simulink model "MCS"  (R2022b)
settings: Solver=FixedStepAuto  StartTime=0.0  StopTime=inf  RelTol=1e-3  EnableMultiTasking=on
undefined symbols (not defined in the file or in its folder): CR, INPUT, LF, MCS_SAMPLING_TIME, SAMPLING_TIME
libraries: instrumentseriallib x2, sharedtransform x2, aerolibanimutils x1, instrumentlib x1
Description:
  | Packet Input/Output
  | 
  | The example model "sldrtex_packetio" shows how to transfer data through
  | UDP communication protocol using binary encoding. The model sends data
  | within one computer, from one UDP port to another. You can modify the
  | model to communicate between two computers by splitting this model
  | into its send and receive parts and running the models on two computers.
  | The yellow blocks are used to send the data, the blue blocks
  | are used to receive the data. Then, please enter the host names or
  | IP addresses of the two computers into the appropriate fields
  | in the Board Setup dialog.
  | 
  | How to run this model in Normal Mode:
  | 
  | 1) Double-click the orange button to switch to Normal Mode if needed.
  | 2) Start the real-time execution using Simulation->Run.
  | 
  | How to run this model in External Mode:
  | 
  | 1) Double-click the orange button to switch to External Mode if needed.
  | 2) Start the real-time execution using Simulation->Run. The model will automatically
  |    build, connect to Simulink in External Mode and start.
settings Model: ExtModeTrigDuration=12000  Creator=The MathWorks, Inc.  LastModifiedBy=drones
settings SolverCC: AlgebraicLoopSolver=TrustRegion
settings DataIOCC: LimitDataPoints=on  SaveFormat=Array  SignalLoggingSaveFormat=ModelDataLogs  ReturnWorkspaceOutputs=off
settings OptimizationCC: ExpressionDepthLimit=2147483647  InitFltsAndDblsToZero=on  EfficientMapNaN2IntZero=off
settings DebuggingCC: MergeDetectMultiDrivingBlocksExec=none  SolverPrmCheckMsg=warning  MultiTaskDSMMsg=none  FcnCallInpInsideContextMsg=warning  UnconnectedInputMsg=warning  UnconnectedOutputMsg=warning  UnconnectedLineMsg=warning  AllowSymbolicDim=off  StateNameClashWarn=warning  SFUnexpectedBacktrackingDiag=warning  SFNoUnconditionalDefaultTransitionDiag=warning  SFExecutionAtInitializationDiag=none  SFMachineParentedDataDiag=warning  ArithmeticOperatorsInVariantConditions=warning
settings HardwareCC: ProdBitPerLong=64  ProdHWDeviceType=Intel->x86-64 (Linux 64)
settings ModelReferenceCC: EnableRefExpFcnMdlSchedulingChecks=on  PropagateSignalLabelsOutOfModel=off
settings SFSimCC: SimUseLocalCustomCode=off  CustomCodeUndefinedFunction=UseInterfaceOnly
settings RTWCC: Description=Simulink Desktop Real-Time  SystemTargetFile=sldrt.tlc  TemplateMakefile=sldrt.tmf  RTWUseLocalCustomCode=off  RTWCompilerOptimization=on  DLArmComputeVersion=19.05
settings CodeAppCC: MaxIdLength=95  StateflowObjectComments=on
settings SimulinkDesktopRealTimeCC: TargetLibSuffix=_sldrt.a  TargetPreCompLibLocation=C:\Program Files\MATLAB\R2022b\toolbox\sldrt\lib\win64  TargetLangStandard=C89/C90 (ANSI)
settings ConfigComp: CovMetricSettings=dsw  CovSaveCumulativeToWorkspaceVar=on  CovSaveSingleToWorkspaceVar=on  CovExternalEMLEnable=off

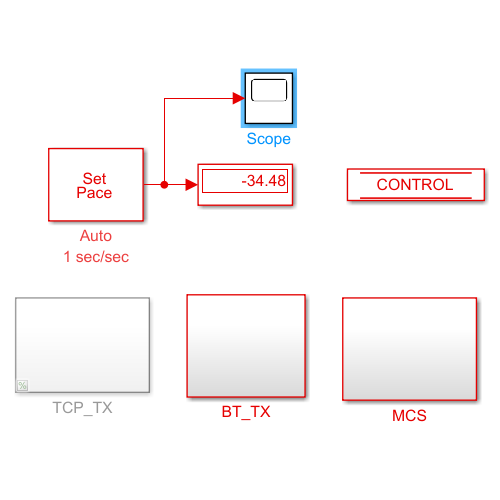
[thumbnail: Simulink's stored preview of the top-level diagram]
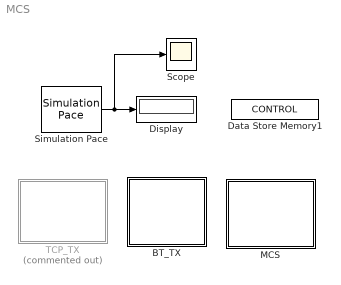
== system MCS ==
  BT_TX : Subsystem
  Data Store Memory1 : DataStoreMemory  Priority=2  DataStoreName=CONTROL  ReadBeforeWriteMsg=warning  WriteAfterWriteMsg=warning  WriteAfterReadMsg=warning  InitialValue=CONTROL_INI  ShowAdditionalParam=off  OutDataTypeStr=Bus: CONTROL_Bus
  Display : Display
  MCS : Subsystem
  Scope : Scope
  Simulation Pace : aerolibanimutils/Simulation Pace  SimulationPace=1  SleepMode=Auto  OutputPaceError=on  SampleTime=MCS_SAMPLING_TIME
  TCP_TX : Subsystem  Commented=on
  wires:
  Simulation Pace/1 -> Scope/1, Display/1

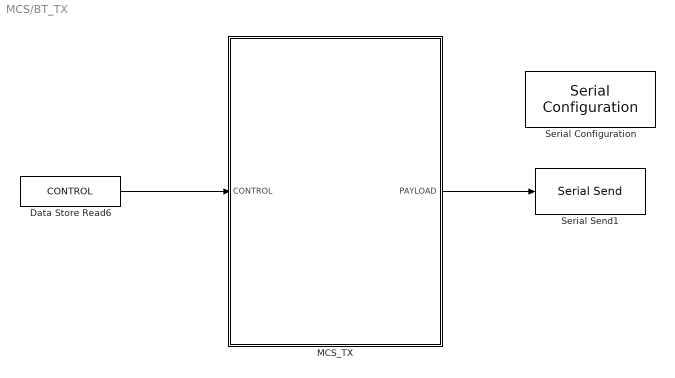
== system MCS/BT_TX ==
  Data Store Read6 : DataStoreRead  DataStoreName=CONTROL  SampleTime=SAMPLING_TIME  IndexOptions=Index vector (dialog)  Indices=1  OutputSizes=1
  MCS_TX : MATLAB Function  Priority=20  TreatAsAtomicUnit=on
  Serial Configuration : instrumentseriallib/Serial Configuration  Priority=-200000  PortSel=COM3  Port=COM3  ComPort=COM3  BaudRate=115200  DataBits=8  Parity=none  StopBits=1  ByteOrder=little-endian  FlowControl=none  Timeout=10e-3  SimulateUsing=Interpreted execution  BlockInModel=on  aMode=1
  Serial Send1 : instrumentseriallib/Serial Send  PortSel=COM3  Port=COM3  ComPort=COM3  Header=[254 ]  Terminator=CR/LF ('\r\n')  CustomTerminator=[]  EnableBlockingMode=off  SimulateUsing=Interpreted execution  BlockInModel=on  aMode=1
  wires:
  Data Store Read6/1 -> MCS_TX/1(CONTROL)
  MCS_TX/1(PAYLOAD) -> Serial Send1/1

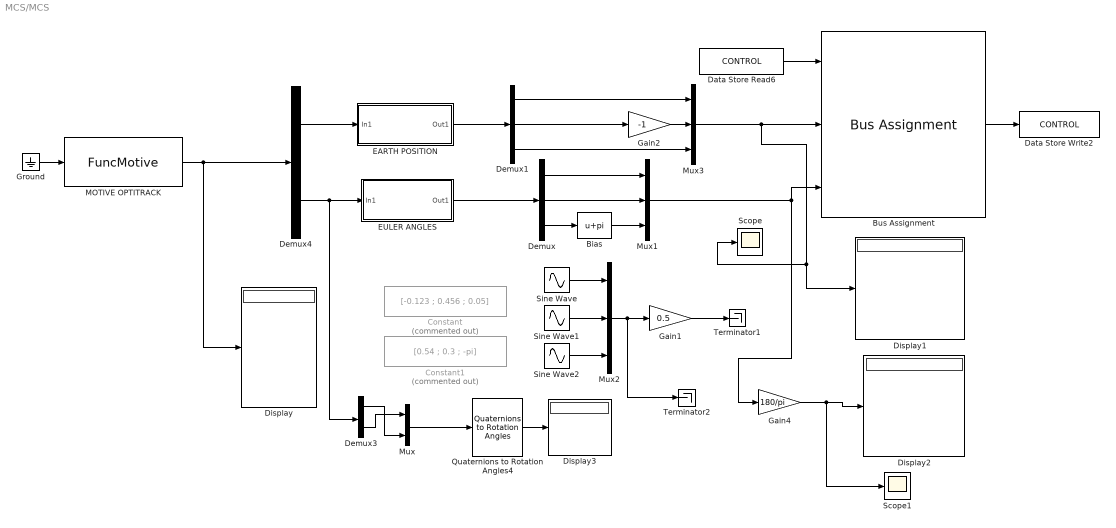
== system MCS/MCS ==
  Bias : Bias  Bias=pi  SaturateOnIntegerOverflow=off
  Bus Assignment : BusAssignment  AssignedSignals=INPUT.MCS_EARTH_POS,INPUT.MCS_EULER_ANG
  Constant : Constant  Commented=on  Value=[-0.123 ; 0.456 ; 0.05]  SampleTime=SAMPLING_TIME
  Constant1 : Constant  Commented=on  Value=[0.54 ; 0.3 ; -pi]  SampleTime=SAMPLING_TIME
  Data Store Read6 : DataStoreRead  DataStoreName=CONTROL  SampleTime=MCS_SAMPLING_TIME  IndexOptions=Index vector (dialog)  Indices=1  OutputSizes=1
  Data Store Write2 : DataStoreWrite  DataStoreName=CONTROL  IndexOptions=Index vector (dialog)  Indices=1  OutputSizes=1
  Demux : Demux  Outputs=3
  Demux1 : Demux  Outputs=3
  Demux3 : Demux  Outputs=[1 -1]
  Demux4 : Demux  Outputs=[3 4]
  Display{,1..3} (4 alike) : Display
  EARTH POSITION : Subsystem
  EULER ANGLES : Subsystem
  Gain1 : Gain  Gain=0.5
  Gain2 : Gain  Gain=-1
  Gain4 : Gain  Gain=180/pi
  Ground : Ground
  MOTIVE OPTITRACK : M-S-Function  FunctionName=FuncMotive  Parameters=1
  Mux : Mux  Inputs=2
  Mux1 : Mux  Inputs=3
  Mux2 : Mux  Inputs=3
  Mux3 : Mux  Inputs=3
  Quaternions to Rotation Angles4 : sharedtransform/Quaternions to Rotation Angles  rotationOrder=YZX  aMode=aMode
  Scope : Scope
  Scope1 : Scope
  Sine Wave : Sin  SineType=Sample based  Amplitude=2  Bias=0.5  Samples=360  SampleTime=MCS_SAMPLING_TIME
  Sine Wave1 : Sin  SineType=Sample based  Amplitude=2  Bias=0.5  Samples=360  SampleTime=MCS_SAMPLING_TIME  Offset=60
  Sine Wave2 : Sin  SineType=Sample based  Amplitude=2  Bias=0.5  Samples=360  SampleTime=MCS_SAMPLING_TIME  Offset=120
  Terminator1 : Terminator
  Terminator2 : Terminator
  wires:
  Ground/1 -> MOTIVE OPTITRACK/1
  Demux4/2 -> Demux3/1, EULER ANGLES/1(In1)
  Demux4/1 -> EARTH POSITION/1(In1)
  Data Store Read6/1 -> Bus Assignment/1
  Bus Assignment/1 -> Data Store Write2/1
  MOTIVE OPTITRACK/1 -> Display/1, Demux4/1
  Demux3/2 -> Mux/1
  Mux/1 -> Quaternions to Rotation Angles4/1
  Quaternions to Rotation Angles4/1 -> Display3/1
  Demux3/1 -> Mux/2
  Demux/3 -> Bias/1
  Bias/1 -> Mux1/3
  Demux/2 -> Mux1/2
  Demux/1 -> Mux1/1
  EULER ANGLES/1(Out1) -> Demux/1
  Sine Wave/1 -> Mux2/1
  Sine Wave1/1 -> Mux2/2
  Sine Wave2/1 -> Mux2/3
  Mux2/1 -> Terminator2/1, Gain1/1
  Gain4/1 -> Scope1/1, Display2/1
  EARTH POSITION/1(Out1) -> Demux1/1
  Gain1/1 -> Terminator1/1
  Mux1/1 -> Gain4/1, Bus Assignment/3
  Mux3/1 -> Scope/1, Display1/1, Bus Assignment/2
  Demux1/1 -> Mux3/1
  Demux1/2 -> Gain2/1
  Gain2/1 -> Mux3/2
  Demux1/3 -> Mux3/3

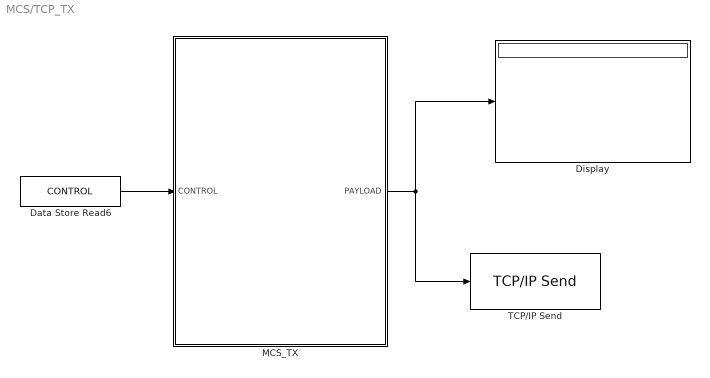
== system MCS/TCP_TX ==
  Data Store Read6 : DataStoreRead  DataStoreName=CONTROL  SampleTime=MCS_SAMPLING_TIME  IndexOptions=Index vector (dialog)  Indices=1  OutputSizes=1
  Display : Display
  MCS_TX : MATLAB Function  Priority=20  TreatAsAtomicUnit=on
  TCP/IP Send : instrumentlib/TCP//IP Send  Host=192.168.0.107  Port=15000  ByteOrder=big-endian  EnableBlockingMode=off  Timeout=SAMPLING_TIME  TransferDelay=off  SimulateUsing=Interpreted execution
  wires:
  MCS_TX/1(PAYLOAD) -> TCP/IP Send/1, Display/1
  Data Store Read6/1 -> MCS_TX/1(CONTROL)

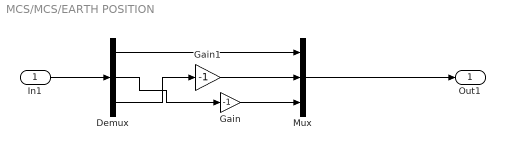
== system MCS/MCS/EARTH POSITION ==
  In1 : Inport
  Demux : Demux  Outputs=3
  Gain : Gain  Gain=-1
  Gain1 : Gain  Gain=-1
  Mux : Mux  Inputs=3
  Out1 : Outport  VectorParamsAs1DForOutWhenUnconnected=off
  wires:
  In1/1 -> Demux/1
  Demux/1 -> Mux/1
  Demux/2 -> Gain/1
  Demux/3 -> Gain1/1
  Mux/1 -> Out1/1
  Gain/1 -> Mux/3
  Gain1/1 -> Mux/2

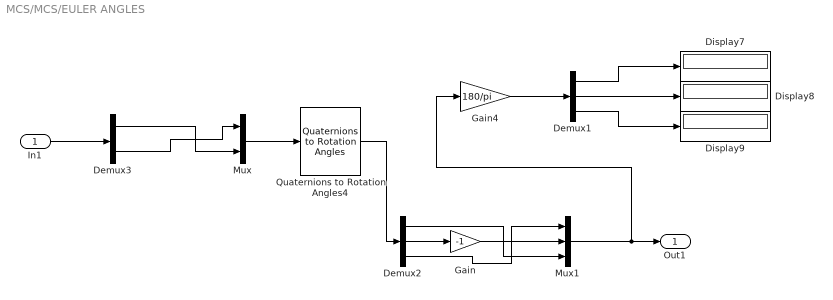
== system MCS/MCS/EULER ANGLES ==
  In1 : Inport
  Demux1 : Demux  Outputs=3
  Demux2 : Demux  Outputs=3
  Demux3 : Demux  Outputs=[1 -1]
  Display7 : Display
  Display8 : Display
  Display9 : Display
  Gain : Gain  Gain=-1
  Gain4 : Gain  Gain=180/pi
  Mux : Mux  Inputs=2
  Mux1 : Mux  Inputs=3
  Quaternions to Rotation Angles4 : sharedtransform/Quaternions to Rotation Angles  rotationOrder=YZX  aMode=aMode
  Out1 : Outport  VectorParamsAs1DForOutWhenUnconnected=off
  wires:
  Mux/1 -> Quaternions to Rotation Angles4/1
  Demux1/1 -> Display7/1
  Quaternions to Rotation Angles4/1 -> Demux2/1
  Demux1/3 -> Display9/1
  Demux1/2 -> Display8/1
  In1/1 -> Demux3/1
  Demux3/1 -> Mux/2
  Demux3/2 -> Mux/1
  Demux2/1 -> Mux1/3
  Mux1/1 -> Gain4/1, Out1/1
  Gain4/1 -> Demux1/1
  Demux2/3 -> Mux1/1
  Demux2/2 -> Gain/1
  Gain/1 -> Mux1/2

== matlab function MCS/TCP_TX/MCS_TX ==
  data: CONTROL input; PAYLOAD output uint8 size=26
function PAYLOAD = MCS_TX(CONTROL)

% Payload definition
PAYLOAD = [typecast(single(CONTROL.INPUT.MCS_EARTH_POS(1)),'uint8')'
    typecast(single(CONTROL.INPUT.MCS_EARTH_POS(2)),'uint8')'
    typecast(single(CONTROL.INPUT.MCS_EARTH_POS(3)),'uint8')'
    typecast(single(CONTROL.INPUT.MCS_EULER_ANG(1)),'uint8')'
    typecast(single(CONTROL.INPUT.MCS_EULER_ANG(2)),'uint8')'
    typecast(single(CONTROL.INPUT.MCS_EULER_ANG(3)),'uint8')'
    uint8(0) ; uint8(0)];
% CRC computation
CRC_VALUE = uint16(65535);
for nn=1:length(PAYLOAD)-2
    TMP = bitxor(uint16(PAYLOAD(nn)),bitand(CRC_VALUE,uint16(255)));
    TMP4 = bitand(bitshift(TMP,4),uint16(255));
    TMP = bitxor(TMP,TMP4);
    TMP8 = bitshift(TMP,8);
    TMP3 = bitshift(TMP,3);
    TMP_4 = bitshift(TMP,-4); 
    CRC_VALUE = bitxor(bitshift(CRC_VALUE,-8),bitxor(TMP8,bitxor(TMP3,TMP_4)));
    CRC_VALUE = bitand(CRC_VALUE,uint16(65535));
end
CRC1 = uint8(bitand(CRC_VALUE,uint16(255)));
CRC2 = uint8(bitand(bitshift(CRC_VALUE,-8),uint16(255)));
PAYLOAD(end-1) = CRC1;
PAYLOAD(end) = CRC2;

return

== matlab function MCS/BT_TX/MCS_TX ==
  data: CONTROL input; PAYLOAD output uint8 size=26
function PAYLOAD = MCS_TX(CONTROL)

% Payload definition
PAYLOAD = [typecast(single(CONTROL.INPUT.MCS_EARTH_POS(1)),'uint8')'
    typecast(single(CONTROL.INPUT.MCS_EARTH_POS(2)),'uint8')'
    typecast(single(CONTROL.INPUT.MCS_EARTH_POS(3)),'uint8')'
    typecast(single(CONTROL.INPUT.MCS_EULER_ANG(1)),'uint8')'
    typecast(single(CONTROL.INPUT.MCS_EULER_ANG(2)),'uint8')'
    typecast(single(CONTROL.INPUT.MCS_EULER_ANG(3)),'uint8')'
    uint8(0) ; uint8(0)];
% CRC computation
CRC_VALUE = uint16(65535);
for nn=1:length(PAYLOAD)-2
    TMP = bitxor(uint16(PAYLOAD(nn)),bitand(CRC_VALUE,uint16(255)));
    TMP4 = bitand(bitshift(TMP,4),uint16(255));
    TMP = bitxor(TMP,TMP4);
    TMP8 = bitshift(TMP,8);
    TMP3 = bitshift(TMP,3);
    TMP_4 = bitshift(TMP,-4); 
    CRC_VALUE = bitxor(bitshift(CRC_VALUE,-8),bitxor(TMP8,bitxor(TMP3,TMP_4)));
    CRC_VALUE = bitand(CRC_VALUE,uint16(65535));
end
CRC1 = uint8(bitand(CRC_VALUE,uint16(255)));
CRC2 = uint8(bitand(bitshift(CRC_VALUE,-8),uint16(255)));
PAYLOAD(end-1) = CRC1;
PAYLOAD(end) = CRC2;

return
